simulink model "Two_Voltage_Ctrl_of_IM"  (R2024a)
settings: Solver=ode23tb  StartTime=0.0  StopTime=10.0  MaxStep=1e-4  RelTol=1e-3
libraries: spsControlledVoltageSourceLib x6, spsAsynchronousMachineSIUnitsLib x2, simulink x2, sps_lib x1
settings Model: Creator=91889  LastModifiedBy=91889

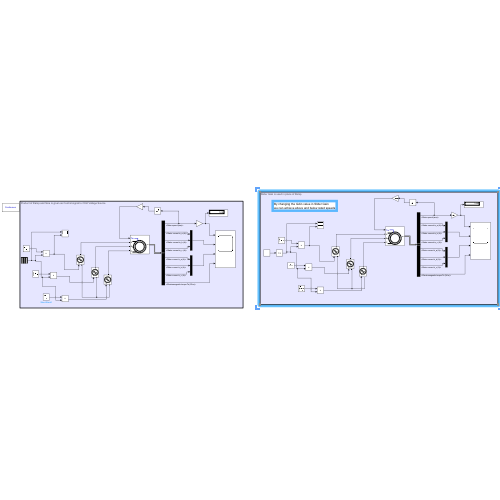
[thumbnail: Simulink's stored preview of the top-level diagram]
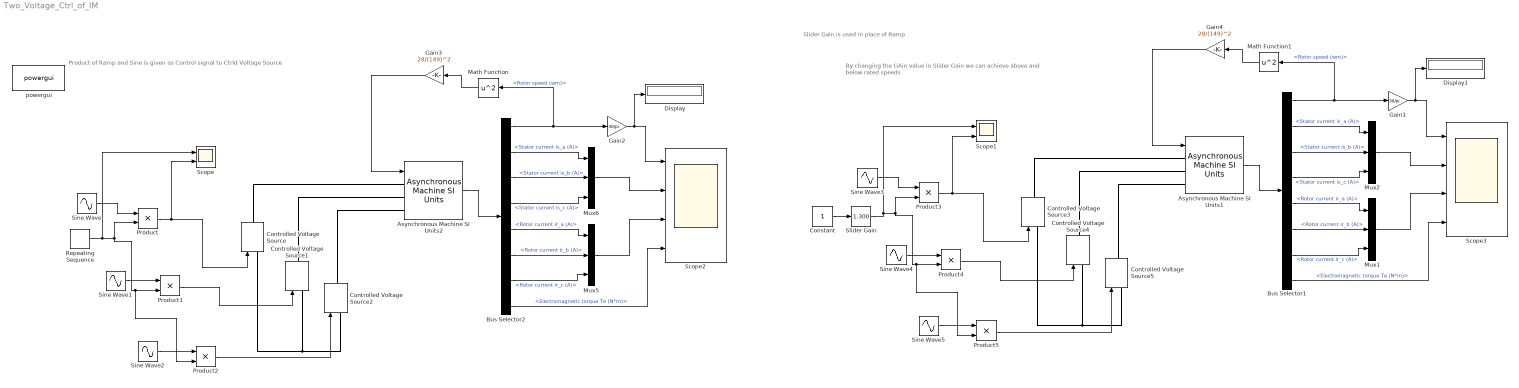
== system Two_Voltage_Ctrl_of_IM ==
  note: By changing the GAin value in Slider Gain
      | we can achieve above and below rated speeds
  note: Slider Gain is used in place of Ramp
  note: Product of Ramp and Sine is given as Control signal to Ctrld Voltage Source
  Asynchronous Machine SI Units1 : spsAsynchronousMachineSIUnitsLib/Asynchronous Machine SI Units  RotorType=Squirrel-cage  PresetModel="15:  5.4 HP (4KW)   400 V  50Hz 1430 RPM"  MechanicalLoad=Torque Tm  ShowDetailedParameters=on  ReferenceFrame=Rotor  Units=SI  MeasurementBus=off  NominalParameters=[4000 400 50]  VoltageRatio=1  Stator=[1.405 0.005839]  Rotor=[1.395 0.005839]  Cage1=[0.4155 0.002066]  Cage2=[0.4168 0.0003495]  Lm=0.1722  Mechanical=[0.0131 0.002985 2]  PolePairs=2  InitialConditions=[0 0 0 0 0 0 0 0]  SimulateSaturation=off  Saturation=[14.03593122, 27.81365428, 53.79336849, 72.68890987, 97.98006896, 148.6815601, 215.7428561, 302.9841135, 428.7778367 ; 230, 322, 414, 460, 506, 552, 598, 644, 690]  LoadFlowParameters=1492000  TsPowergui=0  TsBlock=-1  IterativeModel=Trapezoidal non iterative  IterativeDiscreteModel=Trapezoidal non iterative  Pmec=1.492e+006
  Asynchronous Machine SI Units2 : spsAsynchronousMachineSIUnitsLib/Asynchronous Machine SI Units  RotorType=Squirrel-cage  PresetModel="15:  5.4 HP (4KW)   400 V  50Hz 1430 RPM"  MechanicalLoad=Torque Tm  ShowDetailedParameters=on  ReferenceFrame=Rotor  Units=SI  MeasurementBus=off  NominalParameters=[4000 400 50]  VoltageRatio=1  Stator=[1.405 0.005839]  Rotor=[1.395 0.005839]  Cage1=[0.4155 0.002066]  Cage2=[0.4168 0.0003495]  Lm=0.1722  Mechanical=[0.0131 0.002985 2]  PolePairs=2  InitialConditions=[0 0 0 0 0 0 0 0]  SimulateSaturation=off  Saturation=[14.03593122, 27.81365428, 53.79336849, 72.68890987, 97.98006896, 148.6815601, 215.7428561, 302.9841135, 428.7778367 ; 230, 322, 414, 460, 506, 552, 598, 644, 690]  LoadFlowParameters=1492000  TsPowergui=0  TsBlock=-1  IterativeModel=Trapezoidal non iterative  IterativeDiscreteModel=Trapezoidal non iterative  Pmec=1.492e+006
  Bus Selector1 : BusSelector  OutputSignals=Mechanical.Rotor speed (wm),Stator measurements.Stator current is_a (A),Stator measurements.Stator current is_b (A),Stator measurements.Stator current is_c (A),Rotor measurements.Rotor current ir_a (A),Rotor measurements.Rotor current ir_b (A),Rotor measurements.Rotor current ir_c (A),Mechanical.Electromagnetic torque Te (N*m)
  Bus Selector2 : BusSelector  OutputSignals=Mechanical.Rotor speed (wm),Stator measurements.Stator current is_a (A),Stator measurements.Stator current is_b (A),Stator measurements.Stator current is_c (A),Rotor measurements.Rotor current ir_a (A),Rotor measurements.Rotor current ir_b (A),Rotor measurements.Rotor current ir_c (A),Mechanical.Electromagnetic torque Te (N*m)
  Constant : Constant
  Controlled Voltage Source{,1..5} (6 alike) : spsControlledVoltageSourceLib/Controlled Voltage Source  Initialize=on  Source_Type=AC  Amplitude=0  Phase=0  Frequency=0  Measurements=None
  Display : Display
  Display1 : Display
  Gain1 : Gain  Gain=30/pi
  Gain2 : Gain  Gain=30/pi
  Gain3 : Gain  Gain=28/(149)^2
  Gain4 : Gain  Gain=28/(149)^2
  Math Function : Math  Operator=square
  Math Function1 : Math  Operator=square
  Mux{1..2,5..6} (4 alike) : Mux  Inputs=3
  Product{,1..5} (6 alike) : Product
  Repeating Sequence : simulink/Sources/Repeating Sequence  rep_seq_t=[0 0.2 10]  rep_seq_y=[0 1 1]
  Scope : Scope  NumInputPorts=2
  Scope1 : Scope  NumInputPorts=2
  Scope2 : Scope  NumInputPorts=4
  Scope3 : Scope  NumInputPorts=4
  Sine Wave : Sin  Amplitude=327  Frequency=50*2*pi  SampleTime=0
  Sine Wave1 : Sin  Amplitude=327  Frequency=50*2*pi  Phase=-120*(pi/180)  SampleTime=0
  Sine Wave2 : Sin  Amplitude=327  Frequency=50*2*pi  Phase=120*(pi/180)  SampleTime=0
  Sine Wave3 : Sin  Amplitude=327  Frequency=50*2*pi  SampleTime=0
  Sine Wave4 : Sin  Amplitude=327  Frequency=50*2*pi  Phase=-120*(pi/180)  SampleTime=0
  Sine Wave5 : Sin  Amplitude=327  Frequency=50*2*pi  Phase=120*(pi/180)  SampleTime=0
  Slider Gain : simulink/Math Operations/Slider Gain  gain=1.300  low=0  high=2
  powergui : sps_lib/powergui  Priority=1  SimulationMode=Continuous  SampleTime=50e-6  frequency=60  Iterations=50  frequencyindice=50  Pbase=100e6  ErrMax=1e-4  UnitsV=kV  UnitsW=MW  buscounter=0  FunctionMessages=off  echomessages=off  EnableUseOfTLC=off  CurrentSourceSwitches=off  DisableSnubberDevices=off  DisableRonSwitches=off  DisableVfSwitches=off  DisplayEquations=off  AutomaticDiscreteSolvers=off  SolverType=Tustin/Backward Euler (TBE)  Interpol=off  ExternalGateDelay=off  methode=off  Ts=100  x0status=blocks  SPID=on  SwTol=0  HookPort=off  NonlinearTolerance=1e-4  nMaxIteration=100  ContinueOnMaxIteration=off  RestoreLinks=warning  ResistiveCurrentMeasurement=off  Frange=[0:2:500]  Ylog=off  Xlog=on  ShowGrid=off  save=off  variable=ZData  structure=0  ZoomFFT=off  StartTime=0.0  cycles=1  DisplayStyle=1  fundamental=60  FreqAxis=off  MaxFrequency=1000  frequencyindicesteady=1  RmsSteady=1  display=off
  wires:
  Gain3/1 -> Asynchronous Machine SI Units2/1
  Mux6/1 -> Scope2/2
  Bus Selector2/2 -> Mux6/1  "<Stator current is_a (A)>"
  Asynchronous Machine SI Units2/1 -> Bus Selector2/1
  Bus Selector2/6 -> Mux5/2  "<Rotor current ir_b (A)>"
  Bus Selector2/8 -> Scope2/4  "<Electromagnetic torque Te (N*m)>"
  Gain2/1 -> Display/1, Scope2/1
  Bus Selector2/3 -> Mux6/2  "<Stator current is_b (A)>"
  Bus Selector2/5 -> Mux5/1  "<Rotor current ir_a (A)>"
  Math Function/1 -> Gain3/1
  Mux5/1 -> Scope2/3
  Bus Selector2/4 -> Mux6/3  "<Stator current is_c (A)>"
  Bus Selector2/7 -> Mux5/3  "<Rotor current ir_c (A)>"
  Bus Selector2/1 -> Math Function/1, Gain2/1  "<Rotor speed (wm)>"
  Sine Wave/1 -> Product/1
  Repeating Sequence/1 -> Scope/1, Product/2, Product2/2, Product1/2
  Product/1 -> Scope/2, Controlled Voltage Source/1
  Sine Wave2/1 -> Product2/1
  Sine Wave1/1 -> Product1/1
  Product1/1 -> Controlled Voltage Source1/1
  Product2/1 -> Controlled Voltage Source2/1
  Bus Selector1/1 -> Math Function1/1, Gain1/1  "<Rotor speed (wm)>"
  Bus Selector1/3 -> Mux2/2  "<Stator current is_b (A)>"
  Sine Wave4/1 -> Product4/1
  Bus Selector1/5 -> Mux1/1  "<Rotor current ir_a (A)>"
  Bus Selector1/7 -> Mux1/3  "<Rotor current ir_c (A)>"
  Bus Selector1/8 -> Scope3/4  "<Electromagnetic torque Te (N*m)>"
  Bus Selector1/4 -> Mux2/3  "<Stator current is_c (A)>"
  Mux1/1 -> Scope3/3
  Bus Selector1/6 -> Mux1/2  "<Rotor current ir_b (A)>"
  Math Function1/1 -> Gain4/1
  Gain1/1 -> Display1/1, Scope3/1
  Bus Selector1/2 -> Mux2/1  "<Stator current is_a (A)>"
  Mux2/1 -> Scope3/2
  Asynchronous Machine SI Units1/1 -> Bus Selector1/1
  Gain4/1 -> Asynchronous Machine SI Units1/1
  Product4/1 -> Controlled Voltage Source4/1
  Product5/1 -> Controlled Voltage Source5/1
  Product3/1 -> Scope1/2, Controlled Voltage Source3/1
  Sine Wave5/1 -> Product5/1
  Sine Wave3/1 -> Product3/1
  Slider Gain/1 -> Scope1/1, Product3/2, Product5/2, Product4/2
  Constant/1 -> Slider Gain/1
  connections:
  Controlled Voltage Source/RConn1 -- Asynchronous Machine SI Units2/LConn1
  Asynchronous Machine SI Units2/LConn2 -- Controlled Voltage Source1/RConn1
  Asynchronous Machine SI Units2/LConn3 -- Controlled Voltage Source2/RConn1
  Controlled Voltage Source/LConn1 -- Controlled Voltage Source1/LConn1 -- Controlled Voltage Source2/LConn1
  Controlled Voltage Source3/LConn1 -- Controlled Voltage Source4/LConn1 -- Controlled Voltage Source5/LConn1
  Controlled Voltage Source3/RConn1 -- Asynchronous Machine SI Units1/LConn1
  Asynchronous Machine SI Units1/LConn2 -- Controlled Voltage Source4/RConn1
  Asynchronous Machine SI Units1/LConn3 -- Controlled Voltage Source5/RConn1
